simulink model "jednacina_stanja"  (R2015a)
settings: Solver=FixedStepDiscrete  StartTime=0.0  StopTime=99.0  FixedStep=1  RelTol=1e-3
settings Model: Creator=Bojana Vasic  LastModifiedBy=Bojana Vasic

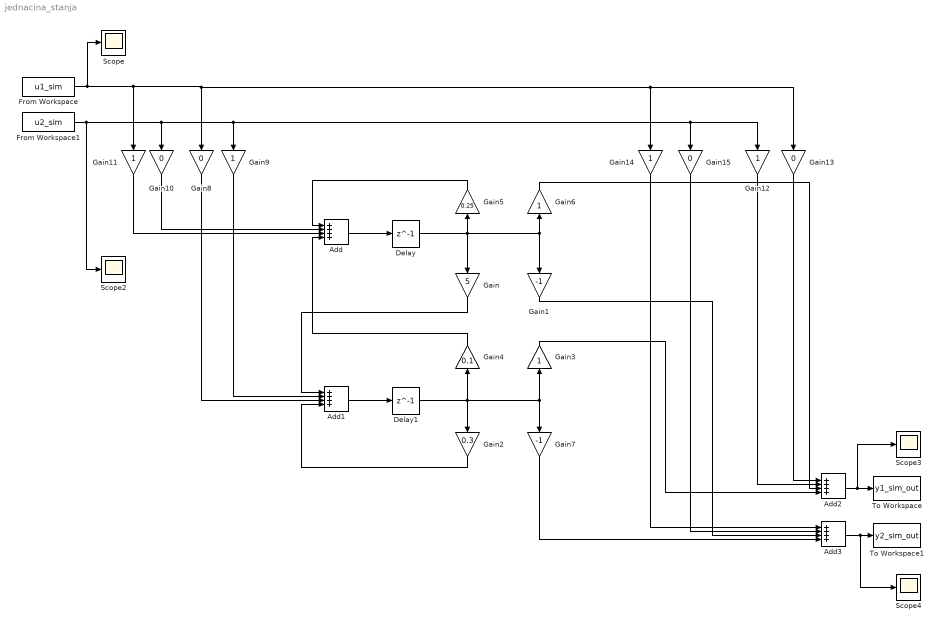
== system jednacina_stanja ==
  Add{,1..3} (4 alike) : Sum  Inputs=++++
  Delay : Delay  DelayLength=1
  Delay1 : Delay  DelayLength=1
  From Workspace : FromWorkspace  VariableName=u1_sim  SampleTime=1
  From Workspace1 : FromWorkspace  VariableName=u2_sim  SampleTime=1
  Gain : Gain  Gain=5
  Gain1 : Gain  Gain=-1
  Gain{8,10,13,15} (4 alike) : Gain  Gain=0
  Gain{3,6,9,11..12,14} (6 alike) : Gain
  Gain2 : Gain  Gain=0.3
  Gain4 : Gain  Gain=0.1
  Gain5 : Gain  Gain=0.25
  Gain7 : Gain  Gain=-1
  Scope{,2..4} (4 alike) : Scope
      Scope2 settings: SaveName=ScopeData2
      Scope3 settings: SaveName=ScopeData3
      Scope4 settings: SaveName=ScopeData4
  To Workspace : ToWorkspace  VariableName=y1_sim_out  SampleTime=-1
      settings: Save2DSignal=2-D array (concatenate along first dimension)
  To Workspace1 : ToWorkspace  VariableName=y2_sim_out  SampleTime=-1
  wires:
  Delay1/1 -> Gain2/1, Gain3/1, Gain7/1, Gain4/1
  Delay/1 -> Gain5/1, Gain/1, Gain1/1, Gain6/1
  Gain5/1 -> Add/1
  Add/1 -> Delay/1
  Gain4/1 -> Add/4
  From Workspace/1 -> Scope/1, Gain14/1, Gain13/1, Gain8/1, Gain11/1
  From Workspace1/1 -> Scope2/1, Gain10/1, Gain15/1, Gain12/1, Gain9/1
  Gain8/1 -> Add1/3
  Gain11/1 -> Add/3
  Gain10/1 -> Add/2
  Gain9/1 -> Add1/2
  Gain/1 -> Add1/1
  Gain2/1 -> Add1/4
  Add1/1 -> Delay1/1
  Gain13/1 -> Add2/1
  Gain12/1 -> Add2/2
  Gain6/1 -> Add2/3
  Gain3/1 -> Add2/4
  Gain1/1 -> Add3/3
  Gain7/1 -> Add3/4
  Gain14/1 -> Add3/1
  Gain15/1 -> Add3/2
  Add2/1 -> Scope3/1, To Workspace/1
  Add3/1 -> Scope4/1, To Workspace1/1
